simulink model "Assembled_scramble"  (R2024b)
settings: Solver=FixedStepAuto  StartTime=0.0  StopTime=10.0  RelTol=1e-3
undefined symbols (not defined in the file): Radix
libraries: androiduilib x3, dspxfrm3 x2, androidaudiovideolib x1, androidcommunicationlib x1, dspsigops x1
settings Model: Creator=hrida  LastModifiedBy=hrida
settings OptimizationCC: DefaultParameterBehavior=Inlined  EnhancedBackFolding=on  PassReuseOutputArgsAs=Individual arguments  ZeroExternalMemoryAtStartup=off  ZeroInternalMemoryAtStartup=off  MaxStackSize=64  OptimizeBlockOrder=speed  DifferentSizesBufferReuse=on  OptimizationCustomize=off  EfficientTunableParamExpr=on
settings DebuggingCC: ParameterTunabilityLossMsg=error
settings HardwareCC: ProdBitPerLong=64  ProdLargestAtomicInteger=LongLong  ProdLargestAtomicFloat=Double  ProdLongLongMode=on  ProdHWDeviceType=ARM Compatible->ARM Cortex-A (64-bit)
settings RTWCC: Description=Embedded Coder  SystemTargetFile=ert.tlc  HardwareBoard=Android Device (64bit)  TLCOptions="-aInlineSetEventsForThisBaseRateFcn=TLC_FALSE -aSuppressMultiTaskScheduler=TLC_FALSE  -aRateBasedStepFcn=0"  TemplateMakefile=ert_default_tmf  GenerateReport=on  RTWVerbose=off  Toolchain=Android SDK/NDK Tools  LaunchReport=on
settings CodeAppCC: ForceParamTrailComments=on  IgnoreCustomStorageClasses=off  OperatorAnnotations=on  SimulinkDataObjDesc=on  SFDataObjDesc=on  InsertBlockDesc=on
settings ERTTargetCC: SupportContinuousTime=on  SupportVariableSizeSignals=on

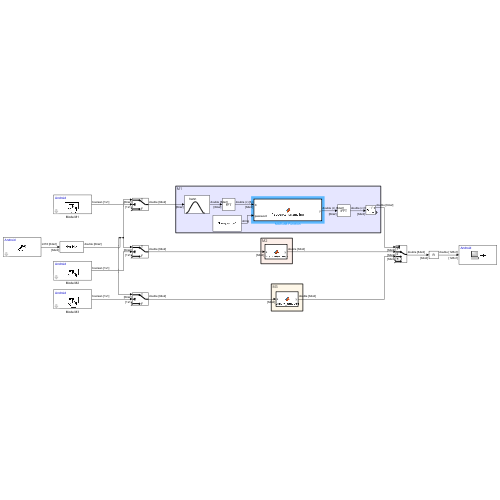
[thumbnail: Simulink's stored preview of the top-level diagram]
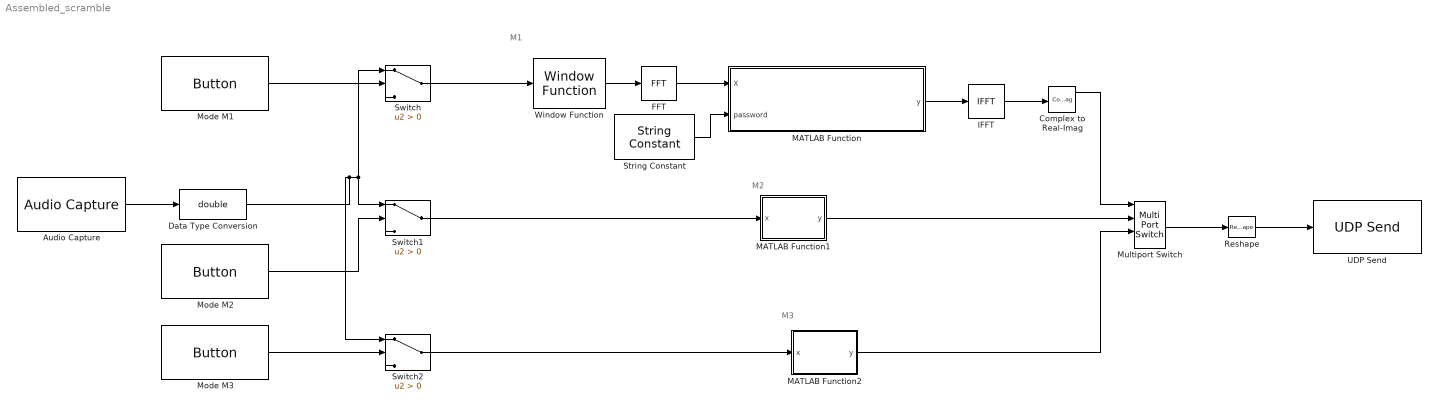
== system Assembled_scramble ==
  note: M3
  note: M2
  note: M1
  Audio Capture : androidaudiovideolib/Audio Capture  SampleFreq=16000  FrameSize=64  SampleTime=0.004  SimulateUsing=Code generation  DeviceStr=0  QueueDuration=0  BlockPlatform=Android  AudioSamplingFreq=44100
  Complex to Real-Imag : ComplexToRealImag
  Data Type Conversion : DataTypeConversion  OutDataTypeStr=double  SaturateOnIntegerOverflow=off  RndMeth=Floor
  FFT : dspxfrm3/FFT  FFTImplementation=Radix-2  CompMethod=Table lookup  TableOpt=NEW  TableOptActive=Speed  BitRevOrder=off  Normalize=off  InheritFFTLength=on  FFTLength=64  WrapInput=on  roundingMode=Ceiling  overflowMode=off  firstCoeffDataTypeStr=Inherit: Same word length as input  firstCoeffLastDataTypeStr=Inherit: Same word length as input  outputMin=[]  outputMax=[]
      settings: LockScale=on
  IFFT : dspxfrm3/IFFT  FFTImplementation=Radix-2  CompMethod=Table lookup  TableOpt=NEW  TableOptActive=Speed  BitRevOrder=off  cs_in=off  Normalize=on  InheritFFTLength=on  FFTLength=64  WrapInput=on  mode=Real  outSamplingMode=Sample based  roundingMode=Ceiling  overflowMode=off  firstCoeffDataTypeStr=Inherit: Same word length as input  firstCoeffLastDataTypeStr=Inherit: Same word length as input  accumDataTypeStr=Inherit: Same as product output  accumLastDataTypeStr=Inherit: Same as product output  outputMin=[]  outputMax=[]
  MATLAB Function : MATLAB Function  TreatAsAtomicUnit=on
  MATLAB Function1 : MATLAB Function  TreatAsAtomicUnit=on
  MATLAB Function2 : MATLAB Function  TreatAsAtomicUnit=on
  Mode M1 : androiduilib/Button  ButtonState=Not pressed  ButtonId=Assembled_scramble/Mode_M1  State=off  SampleTime=0.1  BlockPlatform=Android
  Mode M2 : androiduilib/Button  ButtonState=Not pressed  ButtonId=Assembled_scramble/Mode_M2  State=off  SampleTime=0.1  BlockPlatform=Android
  Mode M3 : androiduilib/Button  ButtonState=Not pressed  ButtonId=Assembled_scramble/Mode_M3  State=off  SampleTime=0.1  BlockPlatform=Android
  Multiport Switch : MultiPortSwitch  DiagnosticForDefault=None  SaturateOnIntegerOverflow=off  InputSameDT=off
  Reshape : Reshape  OutputDimensionality=Customize  OutputDimensions=[128,1]
  String Constant : StringConstant  String="\"Frequency\""
  Switch : Switch  Criteria=u2 > Threshold  SaturateOnIntegerOverflow=off  InputSameDT=off
  Switch1 : Switch  Criteria=u2 > Threshold  SaturateOnIntegerOverflow=off  InputSameDT=off
  Switch2 : Switch  Criteria=u2 > Threshold  SaturateOnIntegerOverflow=off  InputSameDT=off
  UDP Send : androidcommunicationlib/UDP Send  remoteURL='10.7.5.118'  remotePort=25000  localURL='0.0.0.0'  localPortSource=Automatically determine  localPort=-1  sampletime=-1  blockPlatform=Android  separateLengthPort=0
  Window Function : dspsigops/Window Function  winmode=Apply window to input  wintype=Hann  sampmode=Continuous  samptime=1  N=64  Rs=50  beta=10  winsamp=Symmetric  UserWindow=hamming  OptParams=off  UserParams={'symmetric'}  dataType=double  isSigned=on  wordLen=16  udDataType=sfix(16)  fracBitsMode=Best precision  numFracBits=15  roundingMode=Floor  overflowMode=off  numSidelobes=4  sidelobeLevel=-30
  wires:
  Switch2/1 -> MATLAB Function2/1(x)
  Switch1/1 -> MATLAB Function1/1(x)
  Mode M1/1 -> Switch/2
  Switch/1 -> Window Function/1
  Audio Capture/1 -> Data Type Conversion/1
  Mode M3/1 -> Switch2/2
  Mode M2/1 -> Switch1/2
  Window Function/1 -> FFT/1
  FFT/1 -> MATLAB Function/1(X)
  String Constant/1 -> MATLAB Function/2(password)
  MATLAB Function/1(y) -> IFFT/1
  MATLAB Function2/1(y) -> Multiport Switch/3
  MATLAB Function1/1(y) -> Multiport Switch/2
  Multiport Switch/1 -> Reshape/1
  Complex to Real-Imag/1 -> Multiport Switch/1
  IFFT/1 -> Complex to Real-Imag/1
  Data Type Conversion/1 -> Switch1/1, Switch/1, Switch2/1
  Reshape/1 -> UDP Send/1

== matlab function Assembled_scramble/MATLAB Function ==
  data: X input; y output; password input
function y = frequency_scrambling(X,password)

seed=sum(double(char(password)))+length(password);
rng(seed);
key=randperm(31)+1;

y=X;

y(1)=X(1); %DC
y(33)=X(33); %Nyquist

y(2:32)=X(key);
y(34:64)=conj(flipud(y(2:32)));
end

== matlab function Assembled_scramble/MATLAB Function2 ==
  data: x input; y output
function y = watermark_embedding(x)
fs = 16000; % sample rate
N = length(x);
t = (0:N-1)/fs;

% Generate pseudo-random watermark
rng(12345); % fixed seed (same for decryption)
wm = 0.001 * sin(2*pi*3000*t + rand(1,N)); % inaudible high freq tone

% Add watermark
y = x + wm';
end

== matlab function Assembled_scramble/MATLAB Function1 ==
  data: x input; y output
function y = adaptive_noise_masking(x)
% Add adaptive noise shaped to speech spectrum
N = length(x);
X = fft(x);
mag = abs(X);
noise = randn(size(x)); % white noise
NoiseSpec = fft(noise);

% Shape noise based on speech magnitude spectrum
NoiseSpec = NoiseSpec .* (mag ./ max(mag+1e-6));

% Combine signal and shaped noise
Y = X + 0.1 * NoiseSpec; % 0.1 = noise level control
y = real(ifft(Y));
end
